simulink model "FuzzyController"  (R2019a)
settings: Solver=VariableStepAuto  StartTime=0.0  StopTime=20  RelTol=1e-3
undefined symbols (not defined in the file or in its folder): sigbuilder_block
libraries: simulink x2, fuzblock x1
settings Model: Creator=chris  LastModifiedBy=chris

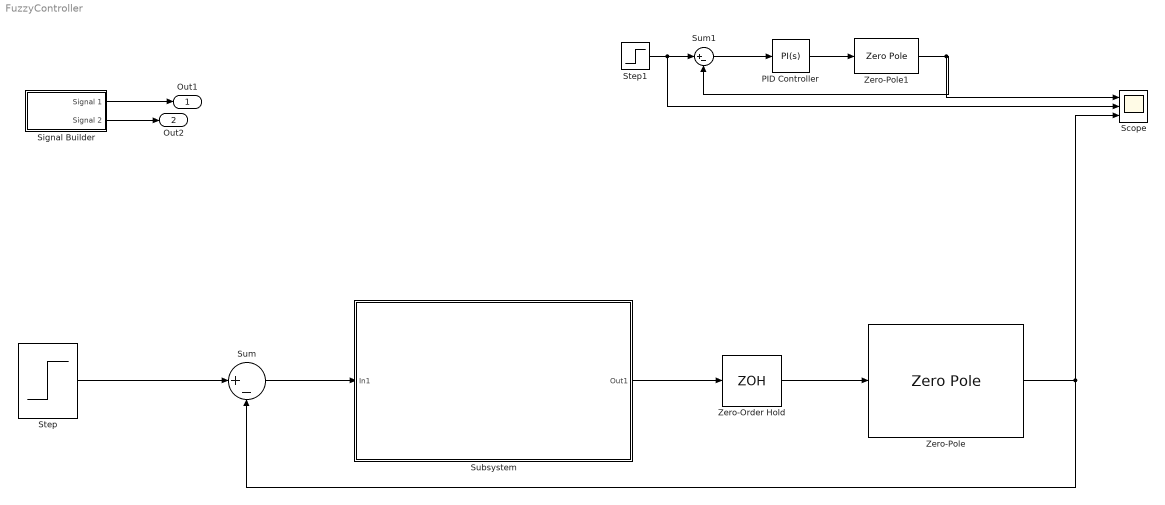
== system FuzzyController ==
  PID Controller : simulink/Continuous/PID Controller  Controller=PI  Form=Parallel  TimeDomain=Continuous-time  SampleTime=-1  IntegratorMethod=Forward Euler  FilterMethod=Forward Euler  ControllerParametersSource=internal  P=1.1  I=0.22  D=0  UseFilter=on  N=100  TunerSelectOption=Transfer Function Based (PID Tuner App)  InitialConditionSource=internal  InitialConditionForIntegrator=0  InitialConditionForFilter=0  DifferentiatorICPrevScaledInput=0  ExternalReset=none  TrackingMode=off  Kt=1  LimitOutput=off  UpperSaturationLimit=inf  LowerSaturationLimit=-inf  LinearizeAsGain=on  AntiWindupMode=none  Kb=1  POutMin=[]  POutMax=[]  IOutMin=[]  IOutMax=[]  DOutMin=[]  DOutMax=[]  NOutMin=[]  NOutMax=[]  SumOutMin=[]  SumOutMax=[]  SaturationOutMin=[]  SaturationOutMax=[]  PParamMin=[]  PParamMax=[]  IParamMin=[]  IParamMax=[]  DParamMin=[]  DParamMax=[]  NParamMin=[]  NParamMax=[]  KbParamMin=[]  KbParamMax=[]  KtParamMin=[]  KtParamMax=[]  KbOutMin=[]  KbOutMax=[]  KtOutMin=[]  KtOutMax=[]  IntegratorOutMin=[]  IntegratorOutMax=[]  FilterOutMin=[]  FilterOutMax=[]  SumI1OutMin=[]  SumI1OutMax=[]  SumI2OutMin=[]  SumI2OutMax=[]  SumI3OutMin=[]  SumI3OutMax=[]  SumI4OutMin=[]  SumI4OutMax=[]  SumDOutMin=[]  SumDOutMax=[]  DifferentiatorOutMin=[]  DifferentiatorOutMax=[]  FilterDiffOutCoefMin=[]  FilterDiffOutCoefMax=[]  ReciprocalOutMin=[]  ReciprocalOutMax=[]  SumDenOutMin=[]  SumDenOutMax=[]  SumNumOutMin=[]  SumNumOutMax=[]  DivideOutMin=[]  DivideOutMax=[]  IntegratorContinuousStateAttributes=''  IntegratorStateMustResolveToSignalObject=off  IntegratorRTWStateStorageClass=Auto  FilterContinuousStateAttributes=''  FilterStateMustResolveToSignalObject=off  FilterRTWStateStorageClass=Auto  ParallelPVariant=InternalParameters  IdealPVariant=Disabled  IVariant=InternalParameters  DVariant=Disabled  IntegratorVariant=Continuous  SatVariant=Disabled  AWVariant=Passthrough  PCopyVariant=Disabled  TRVariant=Disabled  FdbkBlocksVariant=Forward  IdealPFdbkVariant=Disabled  SatFdbkVariant=Disabled  DerivativeFilterVariant=Disabled  NVariant=Disabled  NCopyVariant=Disabled_SignalSpec  FilterICVariant=Disabled  IntegratorICVariant=InternalICs  ExternalResetVariant=Disabled  TRSumVariant=Passthrough  SumFdbkVariant=Disabled  SumVariant=Sum_PI
  Scope : Scope  NumInputPorts=3
  Signal Builder : Subsystem  Tag=STV Subsys  LoadFcn=sigbuilder_block('load');  StartFcn=sigbuilder_block('start');  StopFcn=sigbuilder_block('stop');  ClipboardFcn=sigbuilder_block('clipboard');  mask(Sigbuilder block){tuvar=[0:10]}
      mask help: Simulink:masks:SigbuilderBlock_MD
      mask init:
      | if ~strcmp(get_param(bdroot(gcbh),'SimulationStatus'),'stopped') tuvar = sigbuilder_block('maskInit'); end
      settings: CopyFcn=sigbuilder_block('copy');  DeleteFcn=sigbuilder_block('delete');  ModelCloseFcn=sigbuilder_block('modelClose');  PreSaveFcn=sigbuilder_block('preSave');  PauseFcn=sigbuilder_block('pause');  ContinueFcn=sigbuilder_block('continue');  NameChangeFcn=sigbuilder_block('namechange');  OpenFcn=sigbuilder_block('open',[120.75 207 550.5 399.75 ]);  CloseFcn=sigbuilder_block('close');
      mask Display: plot(0, 0, 100, 100,[2, 2, 32, 32, 2], [68, 8, 8, 68, 68],[32, 2], [38, 38], [32, 19, 2],[53, 60, 44], [32, 17, 17, 2],[16, 16, 31, 31]);txt = getActiveGroup(gcbh);text(2, 100, txt,'verticalAlignment', 'top');
  Step : Step  Time=0  After=50  SampleTime=0.01
  Step1 : Step  Time=0  After=50  SampleTime=0
  Subsystem : Subsystem
  Sum : Sum  Inputs=|+-
  Sum1 : Sum  Inputs=|+-
  Zero-Order Hold : ZeroOrderHold  SampleTime=-1
  Zero-Pole : ZeroPole  Zeros=[]  Poles="[-0.1  -10]"  Gain=25
  Zero-Pole1 : ZeroPole  Zeros=[]  Poles="[-0.1  -10]"  Gain=25
  Out1 : Outport
  Out2 : Outport  Port=2
  wires:
  Zero-Pole/1 -> Scope/3, Sum/2
  Sum/1 -> Subsystem/1(In1)
  Subsystem/1(Out1) -> Zero-Order Hold/1
  Zero-Order Hold/1 -> Zero-Pole/1
  Signal Builder/1(Signal 1) -> Out1/1
  Zero-Pole1/1 -> Scope/1, Sum1/2
  PID Controller/1 -> Zero-Pole1/1
  Sum1/1 -> PID Controller/1
  Step1/1 -> Scope/2, Sum1/1
  Signal Builder/2(Signal 2) -> Out2/1
  Step/1 -> Sum/1

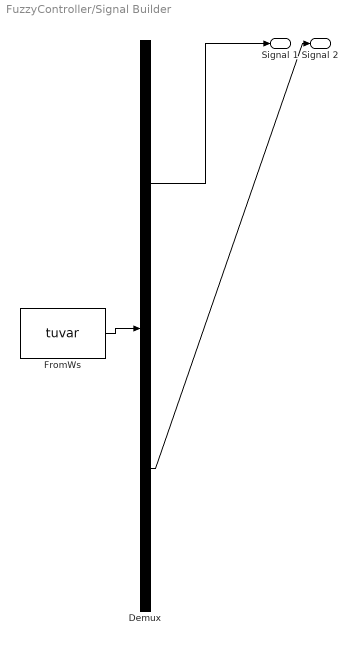
== system FuzzyController/Signal Builder ==
  Demux : Demux  Tag=STV Demux  Outputs=2
  FromWs : FromWorkspace  Tag=STV FromWs  VariableName=tuvar  SampleTime=0
      SigBuilderData=|
      | common.afterFinalStr = 'Extrapolate'
      | common.sampleTime = 0
      | dataSet.timeRange = [0 20]
      | dataSet.name = 'Group 1'
      | sbobj.Groups.Name = 'Group 1'
      | sbobj.Groups.Signals(1).Name = 'Signal 1'
      | sbobj.Groups.Signals(1).XData = [0 5 5 10 10 20]
      | sbobj.Groups.Signals(1).YData = [50 50 20 20 40 40]
      | sbobj.Groups.Signals(2).Name = 'Signal 2'
      | sbobj.Groups.Signals(2).XData = [0 5 10 20]
      | sbobj.Groups.Signals(2).YData = [0 50 50 0]
      | sbobj.Groups.TimeRange = [0 20]
  Signal 1 : Outport  Tag=STV Outport
  Signal 2 : Outport  Tag=STV Outport  Port=2
  wires:
  Demux/1 -> Signal 1/1
  FromWs/1 -> Demux/1
  Demux/2 -> Signal 2/1

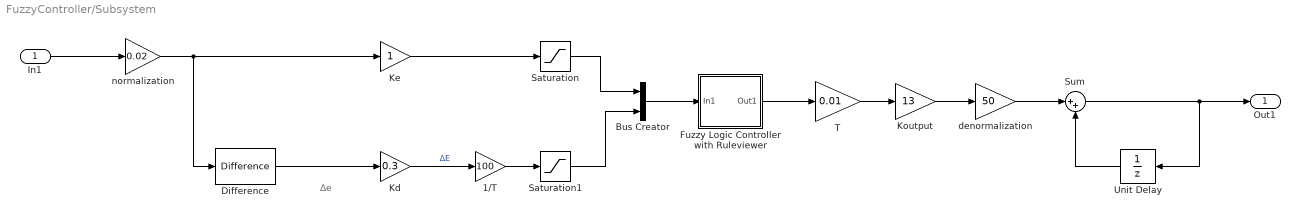
== system FuzzyController/Subsystem ==
  note: Δe
  In1 : Inport
  1/Τ : Gain  Gain=100
  Bus Creator : BusCreator  Inputs=2
  Difference : simulink/Discrete/Difference  ICPrevInput=0.0  OutMin=[]  OutMax=[]  OutDataType=fixdt(1, 16)  OutScaling=2^-10  DoSatur=off
  Fuzzy Logic Controller with Ruleviewer : Subsystem  AncestorBlock=|  mask(Fuzzy Inference System){fismatrix='thecontroller', Ts=0.01}
      | fuzblock/Fuzzy Logic 
      | Controller 
      | with Ruleviewer
      mask prompts: fismatrix "FIS structure:"; Ts "Refresh rate (s):"
      mask help: Fuzzy Inference System (FIS) with a Rule Viewer for fuzzy logic rules.
      mask Help: helpview(fullfile(docroot,'toolbox','fuzzy','fuzzy.map'), 'fuzviewerblock');
      mask DialogControl DescGroupVar Prompt: Fuzzy Inference System
      mask Display: plot(0, -0.3, 6, -0.3, 0, 1.2, 6, 1.2, [0 6], [0 0], [1 2 3],[0 1 0],[2 3 4],[0 1 0],[3 4 5],[0 1 0])
  "Kd " : Gain  Gain=0.3
  "Ke " : Gain
  "Koutput " : Gain  Gain=13
  Saturation : Saturate  UpperLimit=1  LowerLimit=-1
  Saturation1 : Saturate  UpperLimit=1  LowerLimit=-1
  Sum : Sum  Inputs=|++
  T : Gain  Gain=0.01
  Unit Delay : UnitDelay  SampleTime=-1  HasFrameUpgradeWarning=on
  "denormalization " : Gain  Gain=50
  normalization : Gain  Gain=0.02
  Out1 : Outport
  wires:
  Bus Creator/1 -> Fuzzy Logic Controller with Ruleviewer/1(In1)
  normalization/1 -> Difference/1, "Ke "/1
  Unit Delay/1 -> Sum/2
  "Koutput "/1 -> "denormalization "/1
  In1/1 -> normalization/1
  "denormalization "/1 -> Sum/1
  "Ke "/1 -> Saturation/1
  Sum/1 -> Unit Delay/1, Out1/1
  Fuzzy Logic Controller with Ruleviewer/1(Out1) -> T/1
  "Kd "/1 -> 1/Τ/1  "ΔΕ"
  1/Τ/1 -> Saturation1/1
  Saturation/1 -> Bus Creator/1
  T/1 -> "Koutput "/1
  Saturation1/1 -> Bus Creator/2
  Difference/1 -> "Kd "/1

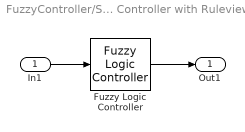
== system FuzzyController/Subsystem/Fuzzy Logic Controller with Ruleviewer ==
  In1 : Inport
  Fuzzy Logic Controller : fuzblock/Fuzzy Logic  Controller  FIS=fismatrix  OutputSampleNumber=101  DataType=double  FuzzifiedInputs=off  RuleFiringStrengths=off  RuleOutputs=off  AggregatedOutputs=off  SimulateUsing=Interpreted execution  OutOfRangeInputValueMessage=warning  NoRuleFiredMessage=warning  EmptyOutputFuzzySetMessage=warning
  Out1 : Outport  InitialOutput=0
  wires:
  Fuzzy Logic Controller/1 -> Out1/1
  In1/1 -> Fuzzy Logic Controller/1
